simulink model "PD"  (R2018b)
settings: Solver=VariableStepAuto  StartTime=0.0  StopTime=10.0  RelTol=1e-3
undefined symbols (not defined in the file): Kd, Kp, parameter_estimated, parameter_true, setpoint
settings Model: Creator=giga4  LastModifiedBy=giga4

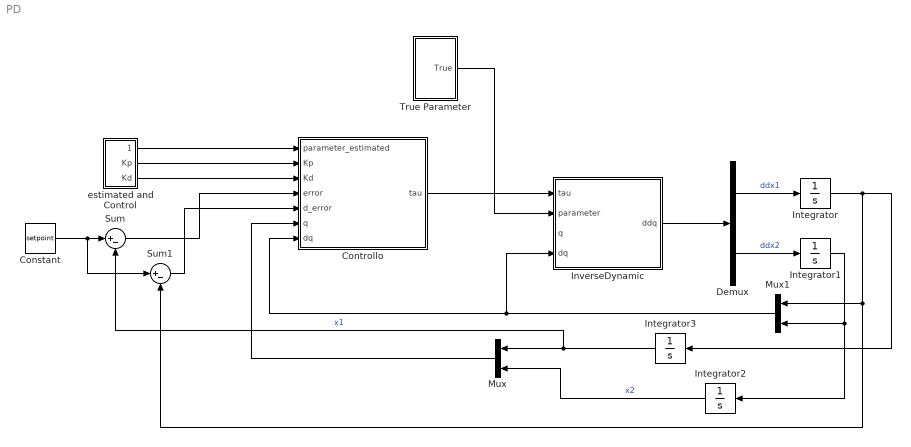
== system PD ==
  Constant : Constant  Value=setpoint
  Controllo : MATLAB Function  TreatAsAtomicUnit=on
  Demux : Demux  Outputs=2
  Integrator{,1..3} (4 alike) : Integrator
  InverseDynamic : MATLAB Function  TreatAsAtomicUnit=on
  Mux : Mux  Inputs=2
  Mux1 : Mux  Inputs=2
  Sum : Sum  Inputs=|+-
  Sum1 : Sum  Inputs=|+-
  True Parameter : Subsystem
  estimated and Control : Subsystem
  wires:
  Controllo/1(tau) -> InverseDynamic/1(tau)
  True Parameter/1(True) -> InverseDynamic/2(parameter)
  estimated and Control/1(Paramter Estimated) -> Controllo/1(parameter_estimated)
  estimated and Control/2(Kp) -> Controllo/2(Kp)
  estimated and Control/3(Kd) -> Controllo/3(Kd)
  InverseDynamic/1(ddq) -> Demux/1
  Demux/1 -> Integrator/1  "ddx1"
  Demux/2 -> Integrator1/1  "ddx2"
  Integrator/1 -> Mux1/1, Sum1/2, Integrator3/1
  Integrator1/1 -> Integrator2/1, Mux1/2
  Integrator3/1 -> Mux/1, Sum/2  "x1"
  Integrator2/1 -> Mux/2  "x2"
  Mux1/1 -> Controllo/7(dq), InverseDynamic/4(dq)
  Constant/1 -> Sum1/1, Sum/1
  Sum/1 -> Controllo/4(error)
  Sum1/1 -> Controllo/5(d_error)
  Mux/1 -> Controllo/6(q)

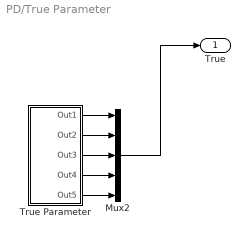
== system PD/True Parameter ==
  Mux2 : Mux  Inputs=5
  True Parameter : Subsystem
  True : Outport
  wires:
  True Parameter/3(Out3) -> Mux2/3
  True Parameter/4(Out4) -> Mux2/4
  True Parameter/5(Out5) -> Mux2/5
  Mux2/1 -> True/1
  True Parameter/1(Out1) -> Mux2/1
  True Parameter/2(Out2) -> Mux2/2

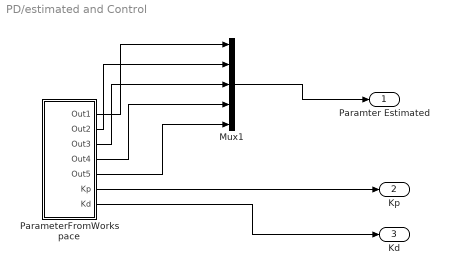
== system PD/estimated and Control ==
  Mux1 : Mux  Inputs=5
  "ParameterFromWorkspace " : Subsystem
  Paramter Estimated : Outport
  Kp : Outport  Port=2
  Kd : Outport  Port=3
  wires:
  "ParameterFromWorkspace "/1(Out1) -> Mux1/1
  "ParameterFromWorkspace "/4(Out4) -> Mux1/4
  "ParameterFromWorkspace "/7(Kd) -> Kd/1
  "ParameterFromWorkspace "/6("Kp ") -> Kp/1
  "ParameterFromWorkspace "/5(Out5) -> Mux1/5
  "ParameterFromWorkspace "/3(Out3) -> Mux1/3
  "ParameterFromWorkspace "/2(Out2) -> Mux1/2
  Mux1/1 -> Paramter Estimated/1

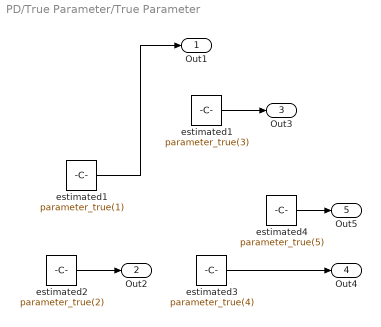
== system PD/True Parameter/True Parameter ==
  estimated1 : Constant  Value=parameter_true(3)
  "estimated1 " : Constant  Value=parameter_true(1)
  estimated2 : Constant  Value=parameter_true(2)
  estimated3 : Constant  Value=parameter_true(4)
  estimated4 : Constant  Value=parameter_true(5)
  Out1 : Outport
  Out2 : Outport  Port=2
  Out3 : Outport  Port=3
  Out4 : Outport  Port=4
  Out5 : Outport  Port=5
  wires:
  "estimated1 "/1 -> Out1/1
  estimated2/1 -> Out2/1
  estimated1/1 -> Out3/1
  estimated4/1 -> Out5/1
  estimated3/1 -> Out4/1

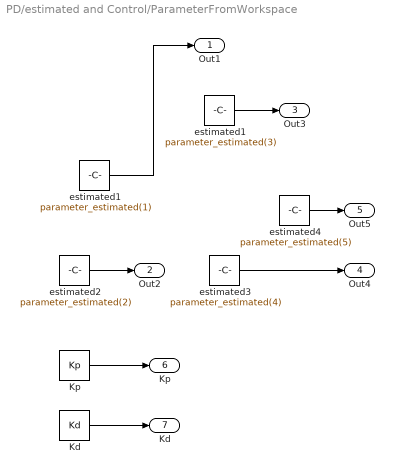
== system PD/estimated and Control/ParameterFromWorkspace  ==
  "Kd " : Constant  Value=Kd
  Kp : Constant  Value=Kp
  estimated1 : Constant  Value=parameter_estimated(3)
  "estimated1 " : Constant  Value=parameter_estimated(1)
  estimated2 : Constant  Value=parameter_estimated(2)
  estimated3 : Constant  Value=parameter_estimated(4)
  estimated4 : Constant  Value=parameter_estimated(5)
  Out1 : Outport
  Out2 : Outport  Port=2
  Out3 : Outport  Port=3
  Out4 : Outport  Port=4
  Out5 : Outport  Port=5
  "Kp " : Outport  Port=6
  Kd : Outport  Port=7
  wires:
  "estimated1 "/1 -> Out1/1
  estimated2/1 -> Out2/1
  estimated1/1 -> Out3/1
  estimated4/1 -> Out5/1
  estimated3/1 -> Out4/1
  Kp/1 -> "Kp "/1
  "Kd "/1 -> Kd/1

== matlab function PD/InverseDynamic ==
  data: tau input; ddq output; parameter input; q input; dq input
function ddq = Inv_Dynamic(tau,parameter,q,dq)

    [B,C,G] = Generatore_Dinamica_SIMULINK(parameter,q,dq);
    
    ddq = B\(tau-C*dq-G); %inv(B)*(tau-C*dq-G);
    
end

== matlab function PD/Controllo ==
  data: parameter_estimated input; Kp input; Kd input; error input; d_error input; tau output; q input; dq input
function tau = PID(parameter_estimated,Kp,Kd,error,d_error,q,dq)


    [B,C,G] = Generatore_Dinamica_SIMULINK(parameter_estimated,q,dq);
   
    
    tau = [0; Kp*error+Kd*d_error+G];

end
